simulink model "IMU_dsPIC_30f4012_LogData_Raw"  (Simulink 7.1)
settings: Solver=FixedStepDiscrete  StartTime=0.0  StopTime=10.0  FixedStep=0.001  RelTol=1e-3
libraries: simulink x9, dsPICdrivers x9
CloseFcn:
  | rtwprivate ssgencode ModelCloseRequest Autopilote_30f4012
settings Model: Creator=Lubin  LastModifiedBy=lubink
settings OptimizationCC: InlineParams=on  OptimizeModelRefInitCode=on  LifeSpan=1
settings DebuggingCC: SaveWithParameterizedLinksMsg=none  MultiTaskDSMMsg=none  MultiTaskCondExecSysMsg=warning
settings HardwareCC: ProdBitPerInt=16  ProdEndianess=LittleEndian  ProdWordSize=16  ProdHWDeviceType=16-bit Generic
settings RTWCC: SystemTargetFile=dspic.tlc  TemplateMakefile=dspic_pic30_gcc.tmf  PostCodeGenCommand=dsPIC_Compile()  Description=Embedded Target for Microchip dsPIC (real-time)  GenerateReport=on  ProcessScript=dspic_make_rtw_hook  IncludeHyperlinkInReport=on  LaunchReport=on  GenerateTraceInfo=on  GenerateTraceReport=on  GenerateTraceReportSl=on  GenerateTraceReportSf=on  GenerateTraceReportEml=on
settings CodeAppCC: IgnoreCustomStorageClasses=off
settings STFCustomTargetCC: ModelReferenceCompliant=off  IncludeMdlTerminateFcn=off  CombineOutputUpdateFcns=on  SuppressErrorStatus=on  ERTCustomFileBanners=on  SupportContinuousTime=off  SupportNonInlinedSFcns=off  SystemTargetFile=dspic.tlc
settings ERTTargetCC: ModelReferenceCompliant=off  CompOptLevelCompliant=off  IncludeMdlTerminateFcn=off  SuppressErrorStatus=on  ERTFirstTimeCompliant=off  ModelStepFunctionPrototypeControlCompliant=off  ExtModeMexFile=ext_serial_win32_comm  InlinedParameterPlacement=NonHierarchical  ERTSrcFileBannerTemplate=dsPIC_code_template.cgt  ERTHdrFileBannerTemplate=dsPIC_code_template.cgt  ERTDataSrcFileTemplate=dsPIC_code_template.cgt  ERTDataHdrFileTemplate=dsPIC_code_template.cgt  ERTCustomFileTemplate=dsPIC_main.tlc
settings CustomProperty: DataType=string  Value=C:\PROGRA~1\MATLAB\R2008a\bin\win32\gmake

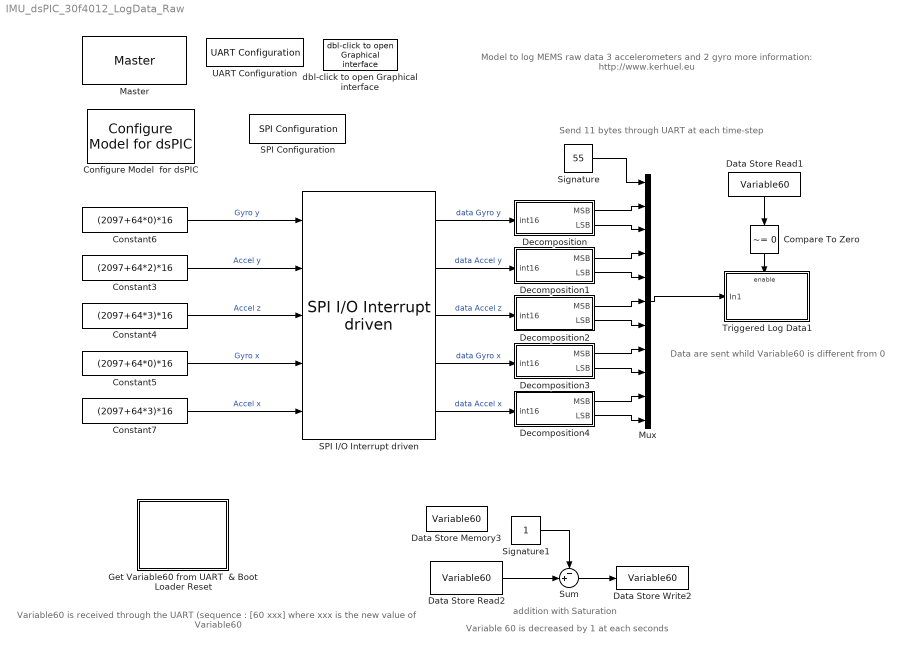
== system IMU_dsPIC_30f4012_LogData_Raw ==
  note: Send 11 bytes through UART at each time-step
  note: Variable 60 is decreased by 1 at each seconds
  note: Data are sent whild Variable60 is different from 0
  note: addition
      | with Saturation
  note: Variable60 is received through the UART
      | (sequence : [60 xxx] where xxx is the new value of Variable60
  note: Model to log MEMS raw data
      | 3 accelerometers and 2 gyro
      | more information: http://www.kerhuel.eu
  Compare To Zero : simulink/Logic and Bit Operations/Compare To Zero  Orientation=down  SystemSampleTime=-1  relop=~=  LogicOutDataTypeMode=boolean  ZeroCross=off
  Configure Model  for dsPIC : dsPICdrivers/Simulink Configuration/Configure Model  for dsPIC
  Constant3 : Constant  Value=(2097+64*2)*16  VectorParams1D=off  OutDataTypeMode=uint16  OutDataType=sfix(16)  OutScaling=2^0  OutDataTypeStr=uint16  SampleTime=-1
  Constant4 : Constant  Value=(2097+64*3)*16  VectorParams1D=off  OutDataTypeMode=uint16  OutDataType=sfix(16)  OutScaling=2^0  OutDataTypeStr=uint16  SampleTime=-1
  Constant5 : Constant  Value=(2097+64*0)*16  VectorParams1D=off  OutDataTypeMode=uint16  OutDataType=sfix(16)  OutScaling=2^0  OutDataTypeStr=uint16  SampleTime=-1
  Constant6 : Constant  Value=(2097+64*0)*16  VectorParams1D=off  OutDataTypeMode=uint16  OutDataType=sfix(16)  OutScaling=2^0  OutDataTypeStr=uint16  SampleTime=-1
  Constant7 : Constant  Value=(2097+64*3)*16  VectorParams1D=off  OutDataTypeMode=uint16  OutDataType=sfix(16)  OutScaling=2^0  OutDataTypeStr=uint16  SampleTime=-1
  Data Store Memory3 : DataStoreMemory  DataStoreName=Variable60  ReadBeforeWriteMsg=warning  WriteAfterWriteMsg=warning  WriteAfterReadMsg=warning  DataType=uint8  OutDataType=sfix(16)  OutScaling=2^0  OutDataTypeStr=uint8
  Data Store Read1 : DataStoreRead  Orientation=down  DataStoreName=Variable60  SampleTime=1
  Data Store Read2 : DataStoreRead  DataStoreName=Variable60  SampleTime=1
  Data Store Write2 : DataStoreWrite  DataStoreName=Variable60  SampleTime=1
  Decomposition : Subsystem
  Decomposition1 : Subsystem
  Decomposition2 : Subsystem
  Decomposition3 : Subsystem
  Decomposition4 : Subsystem
  Get Variable60 from UART  & Boot Loader Reset : Subsystem  AncestorBlock=dsPICdrivers/OTHERS/TinyBld Reset
      mask Display: fprintf('TinyBld\nReset')
  Master : dsPICdrivers/Master  Tag=dsPIC_MASTER  Priority=1  TimeStepType=Timer1  picType=30f4012  fcy=20e6  Quartz_33f=5e6  PLLActive_33f=off  fcyDesired_33f=0  tmr1="[1  19999  0]"  tmr1Info="Time Step : 0.001  ;   Error : 0%  PR1=19999"  tmr2345="[0  0  0  0]"  tmr2345cfg=[-1 -1 -1 -1]  IOautoConf=on  typePort="[ 0   0   0   0   0   0   0   0   0   0   0   0   0   0   0   0   0   0   0   0   0   0   0   0   0   0   0   0   0   0   0   0   0   0   0   0   0   0   0   0   0   0   0   0   0   5   4   0   0   0   0   0   0   0   0   0   0   0   0   0   0   0   0   0   0   0   0  21   0  21   0   0  17   0   0   0   0   0   0   0   0   0   0   0   0   0   0   0   0   0   0   0   0   0   0   0   0   0   0   0   0   0   0   0   0   0   0   0   0   0   0   0 ]"  TRIS="[ 65535  65535  65535  65535  65495  65535  65535 ]"  ADPCFG=0  MasterBusyPort=None  MasterOverloadPort=None  FOSC=XT_PLL8  TempProtection_33f=TEMP_ON  FPBOR=PBOR_OFF  PWRT=PWRT_4  MCLR=MCLR_DIS  PowerSave=off
  Mux : Mux  Inputs=11
  SPI Configuration : dsPICdrivers/SPI PORT/SPI Configuration  Tag=dsPIC_config_SPI  Priority=2  ConfigurationTime=At boot time (only once)  OrderingInOutPopup=None  SampleTime=-1  Frame_Enable=0  Frame_Sync=0  SPI=1  MODE=MASTER  USER_SCALER=96  StartEnable=Enable  SDO_EN=on  DATA_LENGTH=16 bits  SS_EN=off  SMP=Middle of bit  CKP=high  CKE=Idle to Active  Status="Mode 1  -    Fsck= Not Available"
  SPI I/O Interrupt driven : dsPICdrivers/SPI PORT/SPI I//O Interrupt driven  Tag=dsPIC_SPI_IO_Interrupt  SPI=1  nbrTrame=5  mode=read once - interrupt re-enable after block execution  Disable=on  DATA_LENGTH=16 bits  OrderingInOutPopup=None  SampleTime=.001  T1CSL=E5  T1CSH=None  T2CSL=E5  T2CSH=None  T3CSL=E5  T3CSH=None  T4CSL=E3  T4CSH=None  T5CSL=E3  T5CSH=None  T6CSL=None  T6CSH=None  T7CSL=None  T7CSH=None  T8CSL=None  T8CSH=None  T9CSL=None  T9CSH=None  T10CSL=None  T10CSH=None  T11CSL=None  T11CSH=None  T12CSL=None  T12CSH=None  T13CSL=None  T13CSH=None  T14CSL=None  T14CSH=None  T15CSL=None  T15CSH=None
  Signature : Constant  Value=55  OutDataTypeMode=uint8  OutDataType=sfix(16)  OutScaling=2^0  OutDataTypeStr=uint8
  Signature1 : Constant  OutDataTypeMode=uint8  OutDataType=sfix(16)  OutScaling=2^0  OutDataTypeStr=uint8
  Sum : Sum  Inputs=-+|  AccumDataTypeStr=uint16  OutDataTypeMode=uint8  OutDataType=sfix(16)  OutScaling=2^0  OutDataTypeStr=uint8  SampleTime=1  SaturateOnIntegerOverflow=on
  Triggered Log Data1 : Subsystem
  UART Configuration : dsPICdrivers/Serial PORT/UART Configuration  Tag=dsPIC_config_UART  Priority=2  UART=1  proposed_BAUD=115200  ALT_TX_RX=on  InterruptTxWhen=When Transmit Buffer has one empty space (contain 3 characters)  TXInterruptPri=7  TxBufferSize=512  TXEN=on  InterruptRxWhen=When a character is received  RXInterruptPri=1  RxBufferSize=32  BAUD=115200  UxBRG=10  Info="UxBRG = 10   ||  Real Baud : 113636   ||  % error : -1.3573  ||  max 11.3636 Bytes / Step"  RealBaud=0
  dbl-click to open Graphical interface : dsPICdrivers/Serial PORT/dbl-click to open Graphical interface  SystemSampleTime=-1  Nothing=0
  wires:
  Constant6/1 -> SPI I/O Interrupt driven/1  "Gyro y"
  Constant3/1 -> SPI I/O Interrupt driven/2  "Accel y"
  Constant4/1 -> SPI I/O Interrupt driven/3  "Accel z"
  Constant5/1 -> SPI I/O Interrupt driven/4  "Gyro x"
  Constant7/1 -> SPI I/O Interrupt driven/5  "Accel x"
  SPI I/O Interrupt driven/2 -> Decomposition1/1(int16)  "data Accel y"
  SPI I/O Interrupt driven/3 -> Decomposition2/1(int16)  "data Accel z"
  SPI I/O Interrupt driven/4 -> Decomposition3/1(int16)  "data Gyro x"
  SPI I/O Interrupt driven/5 -> Decomposition4/1(int16)  "data Accel x"
  SPI I/O Interrupt driven/1 -> Decomposition/1(int16)  "data Gyro y"
  Signature/1 -> Mux/1
  Decomposition/1(MSB) -> Mux/2
  Decomposition/2(LSB) -> Mux/3
  Decomposition1/1(MSB) -> Mux/4
  Decomposition1/2(LSB) -> Mux/5
  Decomposition2/1(MSB) -> Mux/6
  Decomposition2/2(LSB) -> Mux/7
  Decomposition3/1(MSB) -> Mux/8
  Decomposition3/2(LSB) -> Mux/9
  Decomposition4/1(MSB) -> Mux/10
  Decomposition4/2(LSB) -> Mux/11
  Mux/1 -> Triggered Log Data1/1(In1)
  Data Store Read2/1 -> Sum/2
  Signature1/1 -> Sum/1
  Sum/1 -> Data Store Write2/1
  Compare To Zero/1 -> Triggered Log Data1/Enable
  Data Store Read1/1 -> Compare To Zero/1

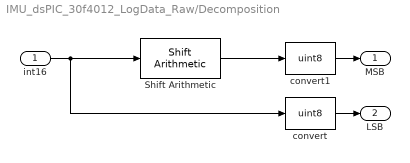
== system IMU_dsPIC_30f4012_LogData_Raw/Decomposition ==
  int16 : Inport
  Shift Arithmetic : simulink/Logic and Bit Operations/Shift Arithmetic  SystemSampleTime=-1  nBitShiftRight=8  nBinPtShiftRight=0
  convert : DataTypeConversion  OutDataTypeMode=uint8  OutDataType=sfix(16)  OutScaling=2^0  OutDataTypeStr=uint8  ConvertRealWorld=Stored Integer (SI)
  convert1 : DataTypeConversion  OutDataTypeMode=uint8  OutDataType=sfix(16)  OutScaling=2^0  OutDataTypeStr=uint8  ConvertRealWorld=Stored Integer (SI)
  MSB : Outport
  LSB : Outport  Port=2
  wires:
  int16/1 -> convert/1, Shift Arithmetic/1
  Shift Arithmetic/1 -> convert1/1
  convert1/1 -> MSB/1
  convert/1 -> LSB/1

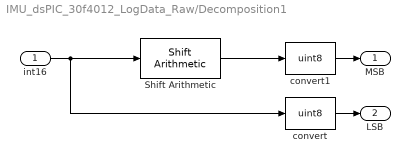
== system IMU_dsPIC_30f4012_LogData_Raw/Decomposition1 ==
  int16 : Inport
  Shift Arithmetic : simulink/Logic and Bit Operations/Shift Arithmetic  SystemSampleTime=-1  nBitShiftRight=8  nBinPtShiftRight=0
  convert : DataTypeConversion  OutDataTypeMode=uint8  OutDataType=sfix(16)  OutScaling=2^0  OutDataTypeStr=uint8  ConvertRealWorld=Stored Integer (SI)
  convert1 : DataTypeConversion  OutDataTypeMode=uint8  OutDataType=sfix(16)  OutScaling=2^0  OutDataTypeStr=uint8  ConvertRealWorld=Stored Integer (SI)
  MSB : Outport
  LSB : Outport  Port=2
  wires:
  convert/1 -> LSB/1
  convert1/1 -> MSB/1
  Shift Arithmetic/1 -> convert1/1
  int16/1 -> Shift Arithmetic/1, convert/1

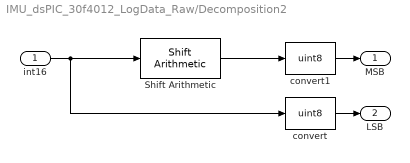
== system IMU_dsPIC_30f4012_LogData_Raw/Decomposition2 ==
  int16 : Inport
  Shift Arithmetic : simulink/Logic and Bit Operations/Shift Arithmetic  SystemSampleTime=-1  nBitShiftRight=8  nBinPtShiftRight=0
  convert : DataTypeConversion  OutDataTypeMode=uint8  OutDataType=sfix(16)  OutScaling=2^0  OutDataTypeStr=uint8  ConvertRealWorld=Stored Integer (SI)
  convert1 : DataTypeConversion  OutDataTypeMode=uint8  OutDataType=sfix(16)  OutScaling=2^0  OutDataTypeStr=uint8  ConvertRealWorld=Stored Integer (SI)
  MSB : Outport
  LSB : Outport  Port=2
  wires:
  int16/1 -> convert/1, Shift Arithmetic/1
  Shift Arithmetic/1 -> convert1/1
  convert1/1 -> MSB/1
  convert/1 -> LSB/1

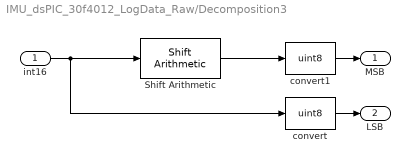
== system IMU_dsPIC_30f4012_LogData_Raw/Decomposition3 ==
  int16 : Inport
  Shift Arithmetic : simulink/Logic and Bit Operations/Shift Arithmetic  SystemSampleTime=-1  nBitShiftRight=8  nBinPtShiftRight=0
  convert : DataTypeConversion  OutDataTypeMode=uint8  OutDataType=sfix(16)  OutScaling=2^0  OutDataTypeStr=uint8  ConvertRealWorld=Stored Integer (SI)
  convert1 : DataTypeConversion  OutDataTypeMode=uint8  OutDataType=sfix(16)  OutScaling=2^0  OutDataTypeStr=uint8  ConvertRealWorld=Stored Integer (SI)
  MSB : Outport
  LSB : Outport  Port=2
  wires:
  convert/1 -> LSB/1
  convert1/1 -> MSB/1
  Shift Arithmetic/1 -> convert1/1
  int16/1 -> Shift Arithmetic/1, convert/1

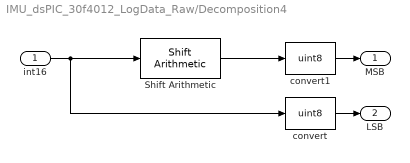
== system IMU_dsPIC_30f4012_LogData_Raw/Decomposition4 ==
  int16 : Inport
  Shift Arithmetic : simulink/Logic and Bit Operations/Shift Arithmetic  SystemSampleTime=-1  nBitShiftRight=8  nBinPtShiftRight=0
  convert : DataTypeConversion  OutDataTypeMode=uint8  OutDataType=sfix(16)  OutScaling=2^0  OutDataTypeStr=uint8  ConvertRealWorld=Stored Integer (SI)
  convert1 : DataTypeConversion  OutDataTypeMode=uint8  OutDataType=sfix(16)  OutScaling=2^0  OutDataTypeStr=uint8  ConvertRealWorld=Stored Integer (SI)
  MSB : Outport
  LSB : Outport  Port=2
  wires:
  int16/1 -> convert/1, Shift Arithmetic/1
  Shift Arithmetic/1 -> convert1/1
  convert1/1 -> MSB/1
  convert/1 -> LSB/1

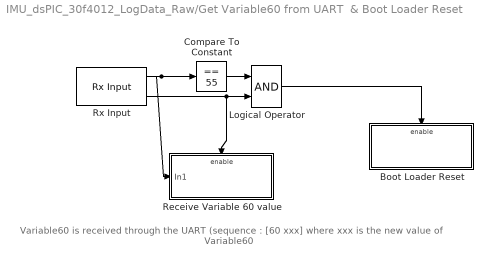
== system IMU_dsPIC_30f4012_LogData_Raw/Get Variable60 from UART  & Boot Loader Reset ==
  note: Variable60 is received through the UART
      | (sequence : [60 xxx] where xxx is the new value of Variable60
  Boot Loader Reset : Subsystem  TreatAsAtomicUnit=on
  Compare To Constant : simulink/Logic and Bit Operations/Compare To Constant  SystemSampleTime=-1  relop===  const=55  LogicOutDataTypeMode=boolean  ZeroCross=off
  Logical Operator : Logic  AllPortsSameDT=off  OutDataTypeMode=boolean  OutDataTypeStr=boolean
  Receive Variable 60 value : Subsystem  TreatAsAtomicUnit=on
  Rx Input : dsPICdrivers/Serial PORT/Rx Input  Tag=dsPIC_RX  Priority=5  UART=1  SampleTime=.01  BlockingFctChk=off  OutputDefault=0  IsPresentFlagChk=on
  wires:
  Rx Input/1 -> Compare To Constant/1, Receive Variable 60 value/1(In1)
  Compare To Constant/1 -> Logical Operator/1
  Rx Input/2 -> Logical Operator/2, Receive Variable 60 value/Enable
  Logical Operator/1 -> Boot Loader Reset/Enable

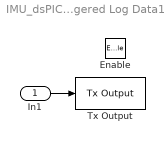
== system IMU_dsPIC_30f4012_LogData_Raw/Triggered Log Data1 ==
  In1 : Inport
  Enable : EnablePort
  Tx Output : dsPICdrivers/Serial PORT/Tx Output  Tag=dsPIC_TX  Priority=5  UART=1  OrderingInOutPopup=None
  wires:
  In1/1 -> Tx Output/1

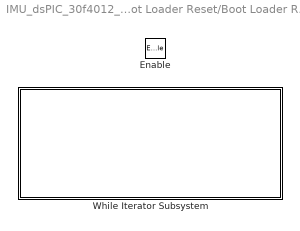
== system IMU_dsPIC_30f4012_LogData_Raw/Get Variable60 from UART  & Boot Loader Reset/Boot Loader Reset ==
  Enable : EnablePort
  While Iterator Subsystem : Subsystem  TreatAsAtomicUnit=on

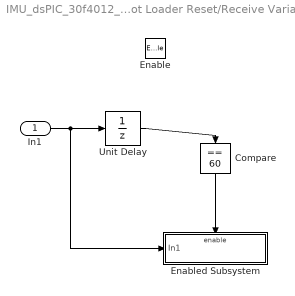
== system IMU_dsPIC_30f4012_LogData_Raw/Get Variable60 from UART  & Boot Loader Reset/Receive Variable 60 value ==
  In1 : Inport  OutDataType=sfix(16)  OutScaling=2^0
  Enable : EnablePort
  Compare : simulink/Logic and Bit Operations/Compare To Constant  Orientation=down  SystemSampleTime=-1  relop===  const=60  LogicOutDataTypeMode=boolean  ZeroCross=off
  Enabled Subsystem : Subsystem  TreatAsAtomicUnit=on
  Unit Delay : UnitDelay  SampleTime=-1
  wires:
  Compare/1 -> Enabled Subsystem/Enable
  Unit Delay/1 -> Compare/1
  In1/1 -> Enabled Subsystem/1(In1), Unit Delay/1

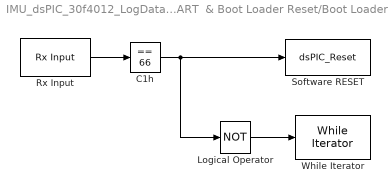
== system IMU_dsPIC_30f4012_LogData_Raw/Get Variable60 from UART  & Boot Loader Reset/Boot Loader Reset/While Iterator Subsystem ==
  C1h : simulink/Logic and Bit Operations/Compare To Constant  SystemSampleTime=-1  relop===  const=66  LogicOutDataTypeMode=boolean  ZeroCross=off
  Logical Operator : Logic  Operator=NOT  AllPortsSameDT=off  OutDataTypeMode=boolean  OutDataTypeStr=boolean
  Rx Input : dsPICdrivers/Serial PORT/Rx Input  Tag=dsPIC_RX  Priority=5  UART=1  SampleTime=-1  BlockingFctChk=on  OutputDefault=0  IsPresentFlagChk=off
  Software RESET : S-Function  Tag=dsPIC_Reset  FunctionName=dsPIC_Reset  EnableBusSupport=off
      mask Description: Reset the microcontroller when input is different from 0
      mask Display:
      | fprintf('Reset');
      | port_label('input', 1 ,'~=0');
  While Iterator : WhileIterator  MaxIters=-1  WhileBlockType=do-while  ResetStates=reset
  wires:
  Logical Operator/1 -> While Iterator/1
  Rx Input/1 -> C1h/1
  C1h/1 -> Software RESET/1, Logical Operator/1

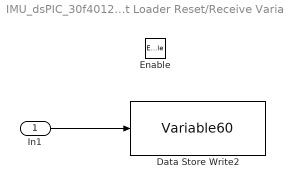
== system IMU_dsPIC_30f4012_LogData_Raw/Get Variable60 from UART  & Boot Loader Reset/Receive Variable 60 value/Enabled Subsystem ==
  In1 : Inport  OutDataType=sfix(16)  OutScaling=2^0
  Enable : EnablePort
  Data Store Write2 : DataStoreWrite  DataStoreName=Variable60  SampleTime=-1
  wires:
  In1/1 -> Data Store Write2/1
